simulink library "avionics_lib"  (Simulink 7.2)
settings: Solver=ode45  SolverMode=SingleTasking  StartTime=0.0  StopTime=10.0  RelTol=1e-3
undefined symbols (not defined in the file or in its folder): AILL, AILLC, AILR, AILRC, alpha_deg, altitude_ft, Ax_g, Ay_g, Az_g, beta_deg, BRAKEC, EGTL, EGTR, ELLIB, ELLIBC, ELLOB, ELLOBC, ELRIB, ELRIBC, ELROB, ELROBC, FLAPLIB, FLAPLIC, FLAPLOB, FLAPLOC, FLAPRIB, FLAPRIC, FLAPROB, FLAPROC, GEARC, KTAS, NAV_altitude_m, NAV_latitude_deg, NAV_longitude_deg, NAV_Ve_mps, NAV_Vn_mps, NAV_Vu_mps, p_deg, phi_deg, psi_deg, q_deg, qbar_psf, r_deg, RPML, RPMR, RUDL, RUDLOC, RUDU, RUDUPC, SPLLIBC, SPLLOBC, SPLRIBC, SPLROBC, STEERC, TEMPAMB_degF, theta_deg, THROTLC, THROTRC
libraries: TransportDelay_lib x5, avionics_lib x1, avionics_T2_lib x1, simulink x1, First_Order_Filter_lib x1
settings Model: Creator=amurch  LastModifiedBy=la1032aw

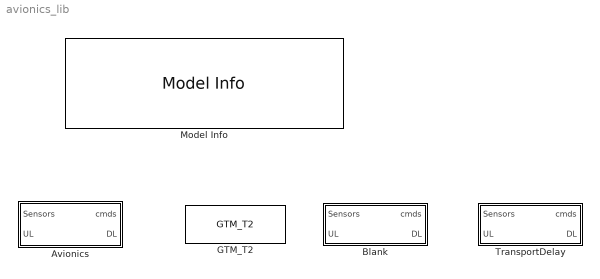
== system avionics_lib ==
  Avionics : Subsystem  BlockChoice=Blank
      settings: TemplateBlock=self  MemberBlocks=Blank,GTM_T2,TransportDelay
  Blank : Subsystem
  GTM_T2 : avionics_T2_lib/GTM_T2  SystemSampleTime=-1
  Model Info : simulink/Model-Wide Utilities/Model Info  SystemSampleTime=-1  InitialBlockCM=None  BlockCM=None  Frame=on  DisplayStringWithTags=|  HorizontalTextAlignment=Center  LeftAlignmentValue=0.5  SourceBlockDiagram=avionics_lib  TagMaxNumber=20
      | Avionics Library
      | %<ModelVersion>
      | Las modified by %<LastModifiedBy> on %<LastModificationDate>
  TransportDelay : Subsystem

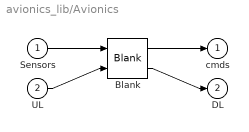
== system avionics_lib/Avionics ==
  Sensors : Inport  OutDataType=sfix(16)  OutScaling=2^0
  UL : Inport  Port=2  OutDataType=sfix(16)  OutScaling=2^0
  Blank : avionics_lib/Blank  SystemSampleTime=-1
  cmds : Outport  OutDataType=sfix(16)  OutScaling=2^0
  DL : Outport  Port=2  OutDataType=sfix(16)  OutScaling=2^0
  wires:
  Sensors/1 -> Blank/1
  UL/1 -> Blank/2
  Blank/1 -> cmds/1
  Blank/2 -> DL/1

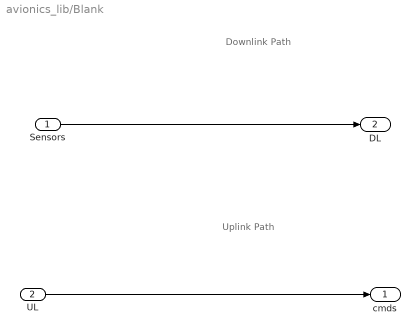
== system avionics_lib/Blank ==
  note: Uplink Path
  note: Downlink Path
  Sensors : Inport  OutDataType=sfix(16)  OutScaling=2^0
  UL : Inport  Port=2  OutDataType=sfix(16)  OutScaling=2^0
  cmds : Outport  OutDataType=sfix(16)  OutScaling=2^0
  DL : Outport  Port=2  OutDataType=sfix(16)  OutScaling=2^0
  wires:
  Sensors/1 -> DL/1
  UL/1 -> cmds/1

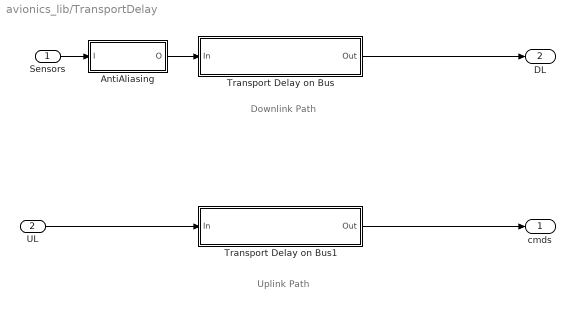
== system avionics_lib/TransportDelay ==
  note: Downlink Path
  note: Uplink Path
  Sensors : Inport  OutDataType=sfix(16)  OutScaling=2^0
  UL : Inport  Port=2  OutDataType=sfix(16)  OutScaling=2^0
  AntiAliasing : Subsystem
  Transport Delay on Bus : Subsystem
  Transport Delay on Bus1 : Subsystem
  cmds : Outport  OutDataType=sfix(16)  OutScaling=2^0
  DL : Outport  Port=2  OutDataType=sfix(16)  OutScaling=2^0
  wires:
  Transport Delay on Bus1/1(Out) -> cmds/1
  Sensors/1 -> AntiAliasing/1(I)
  UL/1 -> Transport Delay on Bus1/1(In)
  Transport Delay on Bus/1(Out) -> DL/1
  AntiAliasing/1(O) -> Transport Delay on Bus/1(In)

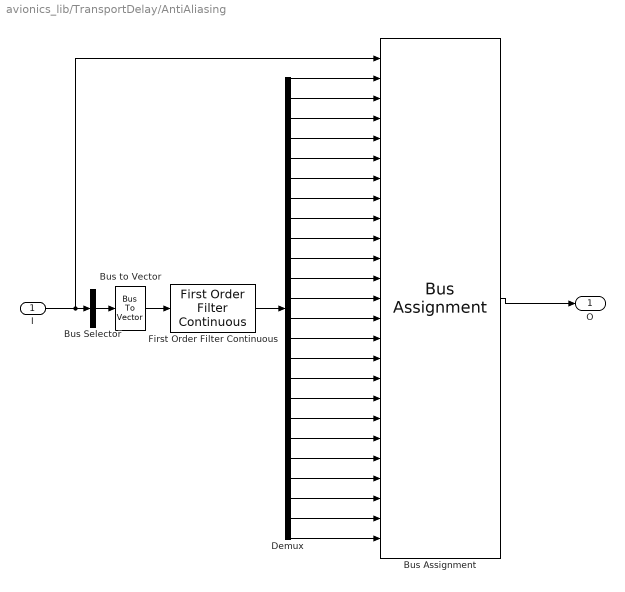
== system avionics_lib/TransportDelay/AntiAliasing ==
  I : Inport  OutDataType=sfix(16)  OutScaling=2^0
  Bus Assignment : BusAssignment  AssignedSignals=AirData.alpha_deg,AirData.beta_deg,AirData.qbar_psf,AirData.KTAS,AirData.TEMPAMB_degF,AirData.altitude_ft,MAG3.p_deg,MAG3.q_deg,MAG3.r_deg,MAG3.Ax_g,MAG3.Ay_g,MAG3.Az_g,SurfacePos.ELLOB,SurfacePos.ELLIB,SurfacePos.ELROB,SurfacePos.ELRIB,SurfacePos.AILL,SurfacePos.AILR,SurfacePos.RUDU,SurfacePos.RUDL,SurfacePos.FLAPLIB,SurfacePos.FLAPLOB,SurfacePos.FLAPRIB,SurfacePos.FLAPROB
  Bus Selector : BusSelector  OutputSignals=AirData.alpha_deg,AirData.beta_deg,AirData.qbar_psf,AirData.KTAS,AirData.TEMPAMB_degF,AirData.altitude_ft,MAG3.p_deg,MAG3.q_deg,MAG3.r_deg,MAG3.Ax_g,MAG3.Ay_g,MAG3.Az_g,SurfacePos.ELLOB,SurfacePos.ELLIB,SurfacePos.ELROB,SurfacePos.ELRIB,SurfacePos.AILL,SurfacePos.AILR,SurfacePos.RUDU,SurfacePos.RUDL,SurfacePos.FLAPLIB,SurfacePos.FLAPLOB,SurfacePos.FLAPRIB,SurfacePos.FLAPROB  OutputAsBus=on
  Bus to Vector : BusToVector
  Demux : Demux  Outputs=24
  First Order Filter Continuous : First_Order_Filter_lib/First Order Filter Continuous  SystemSampleTime=-1  tau=1/2/pi/16
  O : Outport  OutDataType=sfix(16)  OutScaling=2^0
  wires:
  Demux/24 -> Bus Assignment/25
  Demux/23 -> Bus Assignment/24
  Demux/22 -> Bus Assignment/23
  Demux/21 -> Bus Assignment/22
  Demux/20 -> Bus Assignment/21
  Demux/19 -> Bus Assignment/20
  Demux/18 -> Bus Assignment/19
  Demux/17 -> Bus Assignment/18
  Demux/16 -> Bus Assignment/17
  Demux/15 -> Bus Assignment/16
  Demux/14 -> Bus Assignment/15
  Demux/13 -> Bus Assignment/14
  Demux/12 -> Bus Assignment/13
  Demux/11 -> Bus Assignment/12
  Demux/10 -> Bus Assignment/11
  Demux/9 -> Bus Assignment/10
  Demux/8 -> Bus Assignment/9
  Demux/7 -> Bus Assignment/8
  Demux/6 -> Bus Assignment/7
  Demux/5 -> Bus Assignment/6
  Demux/4 -> Bus Assignment/5
  Demux/3 -> Bus Assignment/4
  Demux/2 -> Bus Assignment/3
  Demux/1 -> Bus Assignment/2
  Bus Assignment/1 -> O/1
  First Order Filter Continuous/1 -> Demux/1
  Bus Selector/1 -> Bus to Vector/1
  I/1 -> Bus Assignment/1, Bus Selector/1
  Bus to Vector/1 -> First Order Filter Continuous/1

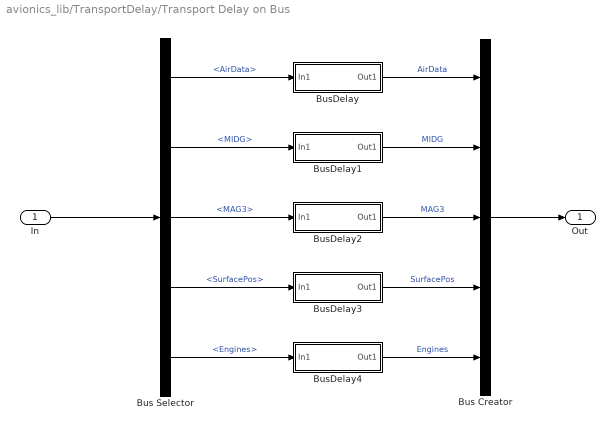
== system avionics_lib/TransportDelay/Transport Delay on Bus ==
  In : Inport
  Bus Creator : BusCreator  Inputs=5
  Bus Selector : BusSelector  OutputSignals=AirData,MIDG,MAG3,SurfacePos,Engines
  BusDelay : Subsystem
  BusDelay1 : Subsystem
  BusDelay2 : Subsystem
  BusDelay3 : Subsystem
  BusDelay4 : Subsystem
  Out : Outport
  wires:
  Bus Creator/1 -> Out/1
  BusDelay4/1(Out1) -> Bus Creator/5  "Engines"
  BusDelay3/1(Out1) -> Bus Creator/4  "SurfacePos"
  BusDelay2/1(Out1) -> Bus Creator/3  "MAG3"
  BusDelay1/1(Out1) -> Bus Creator/2  "MIDG"
  BusDelay/1(Out1) -> Bus Creator/1  "AirData"
  Bus Selector/5 -> BusDelay4/1(In1)  "<Engines>"
  Bus Selector/4 -> BusDelay3/1(In1)  "<SurfacePos>"
  Bus Selector/3 -> BusDelay2/1(In1)  "<MAG3>"
  Bus Selector/2 -> BusDelay1/1(In1)  "<MIDG>"
  Bus Selector/1 -> BusDelay/1(In1)  "<AirData>"
  In/1 -> Bus Selector/1

== system avionics_lib/TransportDelay/Transport Delay on Bus1 ==
  In : Inport
  BusDelay : Subsystem
  Out : Outport
  wires:
  BusDelay/1(Out1) -> Out/1
  In/1 -> BusDelay/1(In1)

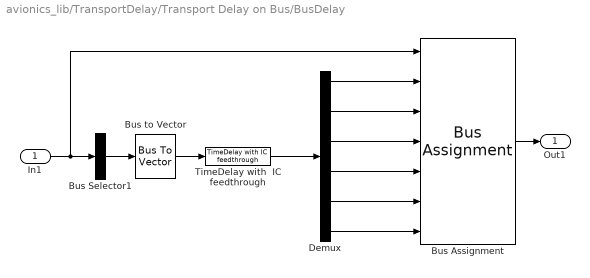
== system avionics_lib/TransportDelay/Transport Delay on Bus/BusDelay ==
  In1 : Inport
  Bus Assignment : BusAssignment  AssignedSignals=alpha_deg,beta_deg,qbar_psf,KTAS,TEMPAMB_degF,altitude_ft
  Bus Selector1 : BusSelector  OutputSignals=alpha_deg,beta_deg,qbar_psf,KTAS,TEMPAMB_degF,altitude_ft  OutputAsBus=on
  Bus to Vector : BusToVector
  Demux : Demux  Outputs=6
  TimeDelay with  IC feedthrough : TransportDelay_lib/TimeDelay with  IC feedthrough  SystemSampleTime=-1  TimeDelay=15e-3
  Out1 : Outport
  wires:
  Bus Assignment/1 -> Out1/1
  Demux/6 -> Bus Assignment/7
  Demux/5 -> Bus Assignment/6
  Demux/4 -> Bus Assignment/5
  Demux/3 -> Bus Assignment/4
  Demux/2 -> Bus Assignment/3
  Demux/1 -> Bus Assignment/2
  TimeDelay with  IC feedthrough/1 -> Demux/1
  Bus to Vector/1 -> TimeDelay with  IC feedthrough/1
  Bus Selector1/1 -> Bus to Vector/1
  In1/1 -> Bus Selector1/1, Bus Assignment/1

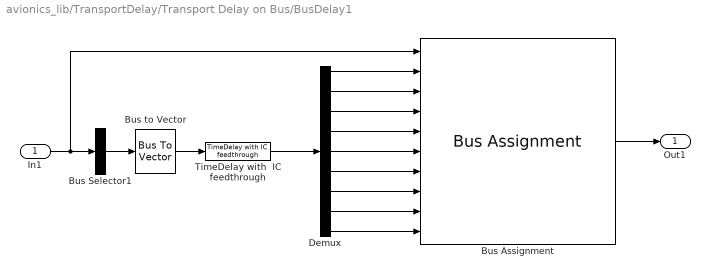
== system avionics_lib/TransportDelay/Transport Delay on Bus/BusDelay1 ==
  In1 : Inport
  Bus Assignment : BusAssignment  AssignedSignals=phi_deg,theta_deg,psi_deg,NAV_latitude_deg,NAV_longitude_deg,NAV_altitude_m,NAV_Vn_mps,NAV_Ve_mps,NAV_Vu_mps
  Bus Selector1 : BusSelector  OutputSignals=phi_deg,theta_deg,psi_deg,NAV_latitude_deg,NAV_longitude_deg,NAV_altitude_m,NAV_Vn_mps,NAV_Ve_mps,NAV_Vu_mps  OutputAsBus=on
  Bus to Vector : BusToVector
  Demux : Demux  Outputs=9
  TimeDelay with  IC feedthrough : TransportDelay_lib/TimeDelay with  IC feedthrough  SystemSampleTime=-1  TimeDelay=15e-3
  Out1 : Outport
  wires:
  Demux/9 -> Bus Assignment/10
  Demux/8 -> Bus Assignment/9
  Demux/7 -> Bus Assignment/8
  Bus Assignment/1 -> Out1/1
  Demux/6 -> Bus Assignment/7
  Demux/5 -> Bus Assignment/6
  Demux/4 -> Bus Assignment/5
  Demux/3 -> Bus Assignment/4
  Demux/2 -> Bus Assignment/3
  Demux/1 -> Bus Assignment/2
  TimeDelay with  IC feedthrough/1 -> Demux/1
  Bus to Vector/1 -> TimeDelay with  IC feedthrough/1
  Bus Selector1/1 -> Bus to Vector/1
  In1/1 -> Bus Selector1/1, Bus Assignment/1

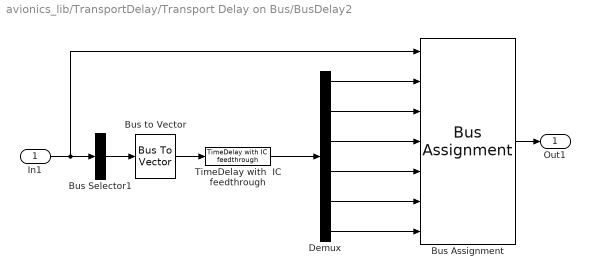
== system avionics_lib/TransportDelay/Transport Delay on Bus/BusDelay2 ==
  In1 : Inport
  Bus Assignment : BusAssignment  AssignedSignals=p_deg,q_deg,r_deg,Ax_g,Ay_g,Az_g
  Bus Selector1 : BusSelector  OutputSignals=p_deg,q_deg,r_deg,Ax_g,Ay_g,Az_g  OutputAsBus=on
  Bus to Vector : BusToVector
  Demux : Demux  Outputs=6
  TimeDelay with  IC feedthrough : TransportDelay_lib/TimeDelay with  IC feedthrough  SystemSampleTime=-1  TimeDelay=15e-3
  Out1 : Outport
  wires:
  Bus Assignment/1 -> Out1/1
  Demux/6 -> Bus Assignment/7
  Demux/5 -> Bus Assignment/6
  Demux/4 -> Bus Assignment/5
  Demux/3 -> Bus Assignment/4
  Demux/2 -> Bus Assignment/3
  Demux/1 -> Bus Assignment/2
  TimeDelay with  IC feedthrough/1 -> Demux/1
  Bus to Vector/1 -> TimeDelay with  IC feedthrough/1
  Bus Selector1/1 -> Bus to Vector/1
  In1/1 -> Bus Selector1/1, Bus Assignment/1

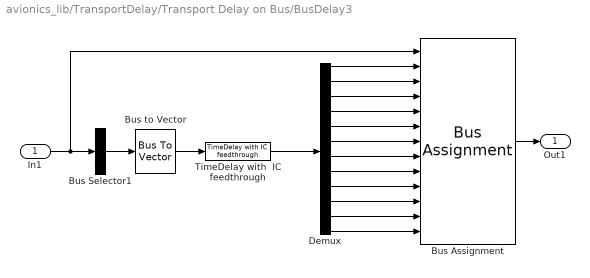
== system avionics_lib/TransportDelay/Transport Delay on Bus/BusDelay3 ==
  In1 : Inport
  Bus Assignment : BusAssignment  AssignedSignals=ELLOB,ELLIB,ELROB,ELRIB,AILL,AILR,RUDU,RUDL,FLAPLIB,FLAPLOB,FLAPRIB,FLAPROB
  Bus Selector1 : BusSelector  OutputSignals=ELLOB,ELLIB,ELROB,ELRIB,AILL,AILR,RUDU,RUDL,FLAPLIB,FLAPLOB,FLAPRIB,FLAPROB  OutputAsBus=on
  Bus to Vector : BusToVector
  Demux : Demux  Outputs=12
  TimeDelay with  IC feedthrough : TransportDelay_lib/TimeDelay with  IC feedthrough  SystemSampleTime=-1  TimeDelay=15e-3
  Out1 : Outport
  wires:
  Demux/12 -> Bus Assignment/13
  Demux/11 -> Bus Assignment/12
  Demux/10 -> Bus Assignment/11
  Demux/9 -> Bus Assignment/10
  Demux/8 -> Bus Assignment/9
  Demux/7 -> Bus Assignment/8
  Demux/6 -> Bus Assignment/7
  Demux/5 -> Bus Assignment/6
  Demux/4 -> Bus Assignment/5
  Demux/3 -> Bus Assignment/4
  Demux/2 -> Bus Assignment/3
  Demux/1 -> Bus Assignment/2
  Bus Assignment/1 -> Out1/1
  TimeDelay with  IC feedthrough/1 -> Demux/1
  Bus to Vector/1 -> TimeDelay with  IC feedthrough/1
  Bus Selector1/1 -> Bus to Vector/1
  In1/1 -> Bus Selector1/1, Bus Assignment/1

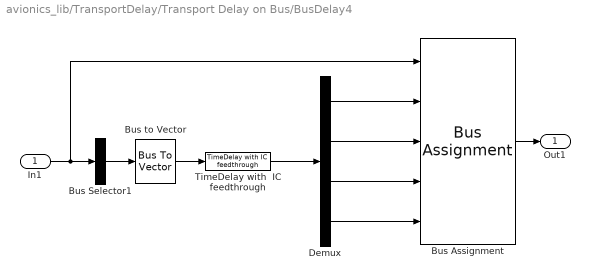
== system avionics_lib/TransportDelay/Transport Delay on Bus/BusDelay4 ==
  In1 : Inport
  Bus Assignment : BusAssignment  AssignedSignals=RPML,EGTL,RPMR,EGTR
  Bus Selector1 : BusSelector  OutputSignals=RPML,EGTL,RPMR,EGTR  OutputAsBus=on
  Bus to Vector : BusToVector
  Demux : Demux
  TimeDelay with  IC feedthrough : TransportDelay_lib/TimeDelay with  IC feedthrough  SystemSampleTime=-1  TimeDelay=15e-3
  Out1 : Outport
  wires:
  Bus Assignment/1 -> Out1/1
  Demux/4 -> Bus Assignment/5
  Demux/3 -> Bus Assignment/4
  Demux/2 -> Bus Assignment/3
  Demux/1 -> Bus Assignment/2
  TimeDelay with  IC feedthrough/1 -> Demux/1
  Bus to Vector/1 -> TimeDelay with  IC feedthrough/1
  Bus Selector1/1 -> Bus to Vector/1
  In1/1 -> Bus Selector1/1, Bus Assignment/1

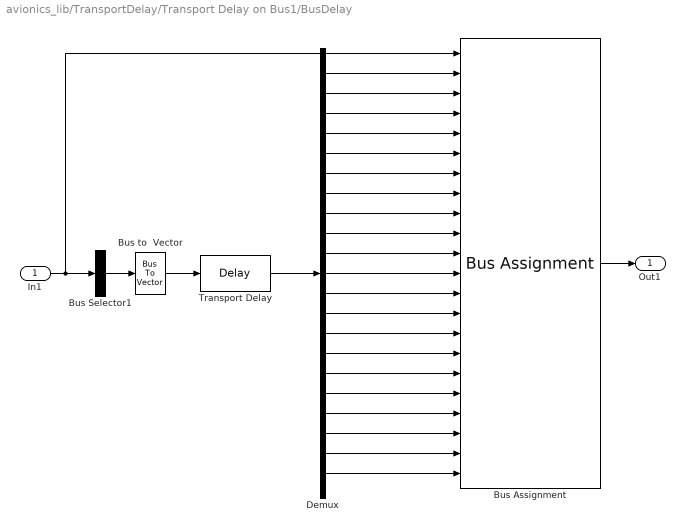
== system avionics_lib/TransportDelay/Transport Delay on Bus1/BusDelay ==
  In1 : Inport
  Bus Assignment : BusAssignment  AssignedSignals=THROTLC,THROTRC,ELLOBC,ELLIBC,ELROBC,ELRIBC,AILLC,AILRC,RUDUPC,RUDLOC,SPLLIBC,SPLLOBC,SPLRIBC,SPLROBC,FLAPLIC,FLAPLOC,FLAPRIC,FLAPROC,GEARC,BRAKEC,STEERC
  Bus Selector1 : BusSelector  OutputSignals=THROTLC,THROTRC,ELLOBC,ELLIBC,ELROBC,ELRIBC,AILLC,AILRC,RUDUPC,RUDLOC,SPLLIBC,SPLLOBC,SPLRIBC,SPLROBC,FLAPLIC,FLAPLOC,FLAPRIC,FLAPROC,GEARC,BRAKEC,STEERC  OutputAsBus=on
  Bus to  Vector : BusToVector
  Demux : Demux  Outputs=21
  Transport Delay : TransportDelay  DelayTime=5e-3
      settings: AttributesFormatString=%<DelayTime>
  Out1 : Outport
  wires:
  Demux/21 -> Bus Assignment/22
  Demux/20 -> Bus Assignment/21
  Demux/19 -> Bus Assignment/20
  Demux/18 -> Bus Assignment/19
  Demux/17 -> Bus Assignment/18
  Demux/16 -> Bus Assignment/17
  Demux/15 -> Bus Assignment/16
  Demux/14 -> Bus Assignment/15
  Demux/13 -> Bus Assignment/14
  Demux/12 -> Bus Assignment/13
  Demux/11 -> Bus Assignment/12
  Demux/10 -> Bus Assignment/11
  Demux/9 -> Bus Assignment/10
  Demux/8 -> Bus Assignment/9
  Demux/7 -> Bus Assignment/8
  Bus Assignment/1 -> Out1/1
  Demux/6 -> Bus Assignment/7
  Demux/5 -> Bus Assignment/6
  Demux/4 -> Bus Assignment/5
  Demux/3 -> Bus Assignment/4
  Demux/2 -> Bus Assignment/3
  Demux/1 -> Bus Assignment/2
  Transport Delay/1 -> Demux/1
  Bus to  Vector/1 -> Transport Delay/1
  Bus Selector1/1 -> Bus to  Vector/1
  In1/1 -> Bus Selector1/1, Bus Assignment/1
